simulink model "ieee9bus_wind_farm"  (R2015b)
settings: Solver=FixedStepAuto  StartTime=0.0  StopTime=40  FixedStep=Ts  RelTol=1e-3
values from neighbouring files (symbols this model uses):
  Cbase = 1/(100*pi*Xbase)    (= 6.0172001169e-06)    [ieee_9.m]
  Lbase = Xbase/(100*pi)    (= 1.68385929791)    [ieee_9.m]
  loadconnection = 15    [ieee_9.m]
  startup = 2    [ieee_9.m]
  Ts = 1e-5    (= 1e-05)    [ieee_9.m]
  Xbase = (Vbase^2)/Sbase    (= 529)    [ieee_9.m]
libraries: powerlib x125, powerlib_meascontrol x23, simulink x10, sps_avr x4, powerlib_extras x1
(part 2 of 2)

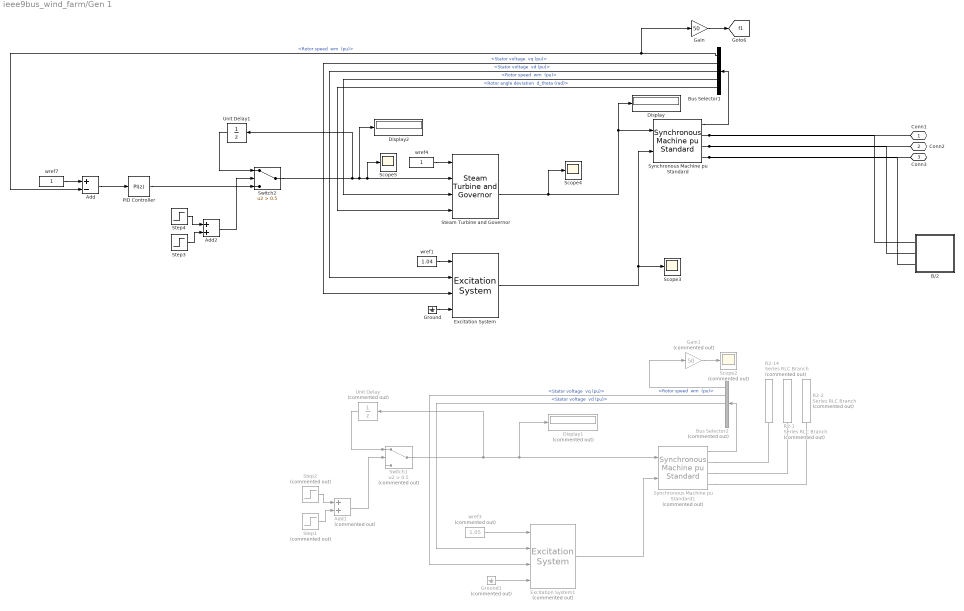
== system ieee9bus_wind_farm/Gen 1 ==
  Add : Sum  Inputs=+-
  Add1 : Sum  Commented=on
  Add2 : Sum
  B/2 : Subsystem
  Bus Selector1 : BusSelector  OutputSignals="Mechanical.Rotor speed  wm  (pu),dq0 components.Stator voltage  vq (pu),dq0 components.Stator voltage  vd (pu),Mechanical.Rotor speed  wm  (pu),Mechanical.Rotor angle deviation  d_theta (rad)"
  Bus Selector2 : BusSelector  Commented=on  OutputSignals="Mechanical.Rotor speed  wm  (pu),dq0 components.Stator voltage  vq (pu),dq0 components.Stator voltage  vd (pu),Mechanical.Rotor speed  wm  (pu),Mechanical.Rotor angle deviation  d_theta (rad)"
  Display : Display
  Display1 : Display  Commented=on
  Display2 : Display
  Excitation System : sps_avr/Excitation System  tr=20e-3  reg=[ 350, 0.001 ]  exc=[ 1, 0 ]  tgr=[ 0, 0 ]  damp=[ 0.001, 0.1 ]  sat=[ 0, 0 ]  lim=[ -11.5, 11.5, 0 ]  v0="[1.0  1.28]"
  Excitation System1 : sps_avr/Excitation System  Commented=on  tr=20e-3  reg=[ 350, 0.001 ]  exc=[ 1, 0 ]  tgr=[ 0, 0 ]  damp=[ 0.001, 0.1 ]  sat=[ 0, 0 ]  lim=[ -11.5, 11.5, 0 ]  v0="[1.0  1.28]"
  Gain : Gain  Gain=50
  Gain1 : Gain  Commented=on  Gain=50
  Ground : Ground
  Ground1 : Ground  Commented=on
  PID Controller : simulink/Continuous/PID Controller  Controller=PI  TimeDomain=Discrete-time  SampleTime=Ts  IntegratorMethod=Forward Euler  FilterMethod=Forward Euler  Form=Parallel  UseFilter=on  ControllerParametersSource=internal  P=1  I=2.5  D=0  N=100  InitialConditionSource=internal  InitialConditionForIntegrator=70/247.5  InitialConditionForFilter=0  ExternalReset=none  LimitOutput=on  UpperSaturationLimit=1  LowerSaturationLimit=1e-6  LinearizeAsGain=on  AntiWindupMode=none  Kb=1  TrackingMode=off  Kt=1  PParamMin=[]  PParamMax=[]  IParamMin=[]  IParamMax=[]  DParamMin=[]  DParamMax=[]  NParamMin=[]  NParamMax=[]  KbParamMin=[]  KbParamMax=[]  KtParamMin=[]  KtParamMax=[]  POutMin=[]  POutMax=[]  IOutMin=[]  IOutMax=[]  DOutMin=[]  DOutMax=[]  NOutMin=[]  NOutMax=[]  KbOutMin=[]  KbOutMax=[]  KtOutMin=[]  KtOutMax=[]  IntegratorOutMin=[]  IntegratorOutMax=[]  FilterOutMin=[]  FilterOutMax=[]  SumOutMin=[]  SumOutMax=[]  SumI1OutMin=[]  SumI1OutMax=[]  SumI2OutMin=[]  SumI2OutMax=[]  SumI3OutMin=[]  SumI3OutMax=[]  SumDOutMin=[]  SumDOutMax=[]  SaturationOutMin=[]  SaturationOutMax=[]  IntegratorContinuousStateAttributes=''  IntegratorStateMustResolveToSignalObject=off  IntegratorRTWStateStorageClass=Auto  FilterContinuousStateAttributes=''  FilterStateMustResolveToSignalObject=off  FilterRTWStateStorageClass=Auto  DifferentiatorICPrevScaledInput=0  DifferentiatorOutMin=[]  DifferentiatorOutMax=[]
  R2-1 : powerlib/Elements/Series RLC Branch  Commented=on  LConnTagsString=__new0  RConnTagsString=__new0  BranchType=R  Resistance=0.0000001  Inductance=0.3*Xbase  SetiL0=off  InitialCurrent=0  Capacitance=1e-6  Setx0=off  InitialVoltage=0  Measurements=None
  R2-14 : powerlib/Elements/Series RLC Branch  Commented=on  LConnTagsString=__new0  RConnTagsString=__new0  BranchType=R  Resistance=0.0000001  Inductance=0.3*Xbase  SetiL0=off  InitialCurrent=0  Capacitance=1e-6  Setx0=off  InitialVoltage=0  Measurements=None
  R2-2 : powerlib/Elements/Series RLC Branch  Commented=on  LConnTagsString=__new0  RConnTagsString=__new0  BranchType=R  Resistance=0.0000001  Inductance=0.3*Xbase  SetiL0=off  InitialCurrent=0  Capacitance=1e-6  Setx0=off  InitialVoltage=0  Measurements=None
  Scope2 : Scope  Commented=on
  Scope3 : Scope
  Scope4 : Scope
  Scope5 : Scope
  Steam Turbine and Governor : powerlib/Machines/Steam Turbine and Governor  gentype=Tandem-compound (multi-mass)  reg1="[ 1  0.05    0 ]"  reg2="[ 0.001  0.3 ]"  reg3="[ -0.1  0.1  0  4.496]"  N=1500  turb1="[ 0  10   3.3   0.5   ]"  turb2="[ 0.5   0.5   0  0 ]"  HA="[  1.5498   0.24894  0  0 ]"  KA="[  83.47  42.702  0  0 ]"  DA="[  0.3104  0.05  0  0 ]*8"  ini1=250.35/555  ini2=[0.5,-120.13]
  Step1 : Step  Commented=on  Time=loadconnection-1  SampleTime=Ts
  Step2 : Step  Commented=on  Time=startup  Before=1  After=0  SampleTime=Ts
  Step3 : Step  Time=loadconnection-1  SampleTime=Ts
  Step4 : Step  Time=startup-2  Before=1  After=0  SampleTime=Ts
  Switch1 : Switch  Commented=on  Criteria=u2 > Threshold  Threshold=0.5
  Switch2 : Switch  Criteria=u2 > Threshold  Threshold=0.5
  Synchronous Machine pu Standard : powerlib/Machines/Synchronous Machine pu Standard  PresetModel=No  MechanicalLoad=Mechanical power Pm  ShowDetailedParameters=on  RotorType=Salient-pole  Units=per unit standard parameters  MeasurementBus=off  NominalParameters=[247.5e+06 16.5e3 50]  Reactances1=[ 1.81, 0.15048, 0.1, 1.76, 0.65, 0.25, 0.15 ]  Reactances2=[0.36135 0.15048 0.1 0.2398275 0.1 0.08316]  dAxisTimeConstants=Short-circuit  qAxisTimeConstants=Short-circuit  TimeConstants1="[ 4.4849  0.0681  0.1  ]"  TimeConstants2=[ 8.0, 0.03, 1.0, 0.07 ]  TimeConstants3="[  4.49  0.0681  0.0513  ]"  TimeConstants4=[ 8.0, 0.03, 0.3371, 0.0295 ]  TimeConstants5=[ 1.01, 0.053, 0.1 ]  TimeConstants6=[ 1.3201, 0.023, 1.0, 0.07 ]  TimeConstants7=[8.96 0.075 0.15]  TimeConstants8=[ 1.3201, 0.0231, 0.3371, 0.0295 ]  StatorResistance=0.00000001  Mechanical=[9.55 0.02056 4]  PolePairs=20  InitialConditions="[ 0  0  0  0  0  0  0  0  1 ]"  SetSaturation=off  Saturation=[0.6404,0.7127,0.8441,0.9214,0.9956,1.082,1.19,1.316,1.457;0.7,0.7698,0.8872,0.9466,0.9969,1.046,1.1,1.151,1.201]  LoadFlowParameters=[1,0,0,0,0]  TsPowergui=0  TsBlock=-1  IterativeModel=Trapezoidal non iterative  BusType=swing  Pref=0  Qref=0  Qmin=-inf  Qmax=inf  PLF=0  QLF=0
  Synchronous Machine pu Standard1 : powerlib/Machines/Synchronous Machine pu Standard  Commented=on  PresetModel=No  MechanicalLoad=Mechanical power Pm  ShowDetailedParameters=on  RotorType=Round  Units=per unit standard parameters  MeasurementBus=off  NominalParameters=[25e+06 16.5e3 50]  Reactances1=[ 1.81, 0.3, 0.23, 1.76, 0.65, 0.25, 0.15 ]  Reactances2=[2.24 0.17 0.12 1.02 0.13 0.08]  dAxisTimeConstants=Short-circuit  qAxisTimeConstants=Short-circuit  TimeConstants1="[ 4.4849  0.0681  0.1  ]"  TimeConstants2=[ 8.0, 0.03, 1.0, 0.07 ]  TimeConstants3="[  4.49  0.0681  0.0513  ]"  TimeConstants4=[ 8.0, 0.03, 0.3371, 0.0295 ]  TimeConstants5=[ 1.01, 0.053, 0.1 ]  TimeConstants6=[ 1.3201, 0.023, 1.0, 0.07 ]  TimeConstants7=[0.012 0.003 0.003]  TimeConstants8=[ 1.3201, 0.0231, 0.3371, 0.0295 ]  StatorResistance=0.0000107875  Mechanical=[2 0.02056 4]  PolePairs=20  InitialConditions="[ 0  0  0  0  0  0  0  0  1 ]"  SetSaturation=off  Saturation=[0.6404,0.7127,0.8441,0.9214,0.9956,1.082,1.19,1.316,1.457;0.7,0.7698,0.8872,0.9466,0.9969,1.046,1.1,1.151,1.201]  LoadFlowParameters=[1,0,0,0,0]  TsPowergui=0  TsBlock=-1  IterativeModel=Trapezoidal non iterative  BusType=swing  Pref=0  Qref=0  Qmin=-inf  Qmax=inf  PLF=0  QLF=0
  Unit Delay : UnitDelay  Commented=on  SampleTime=Ts
  Unit Delay1 : UnitDelay  SampleTime=Ts
  wref1 : Constant  Value=1.04
  wref3 : Constant  Commented=on  Value=1.05
  wref4 : Constant
  wref7 : Constant
  Conn1 : PMIOPort  Port=1  Side=Right
  Conn2 : PMIOPort  Port=2  Side=Right
  Conn3 : PMIOPort  Port=3  Side=Right
  tag scope: f1=global
  wires:
  Synchronous Machine pu Standard/1 -> Bus Selector1/1
  wref1/1 -> Excitation System/1
  Ground/1 -> Excitation System/4
  Excitation System/1 -> Synchronous Machine pu Standard/2, Scope3/1
  Bus Selector1/3 -> Excitation System/2  "<Stator voltage  vd (pu)>"
  Bus Selector1/1 -> Add/2, Gain/1  "<Rotor speed  wm  (pu)>"
  Bus Selector1/2 -> Excitation System/3  "<Stator voltage  vq (pu)>"
  Gain/1 -> [f1]
  Bus Selector1/4 -> Steam Turbine and Governor/3  "<Rotor speed  wm  (pu)>"
  wref4/1 -> Steam Turbine and Governor/1
  Bus Selector1/5 -> Steam Turbine and Governor/4  "<Rotor angle deviation  d_theta (rad)>"
  Steam Turbine and Governor/3 -> Scope4/1, Display/1, Synchronous Machine pu Standard/1
  Synchronous Machine pu Standard1/1 -> Bus Selector2/1
  wref3/1 -> Excitation System1/1
  Ground1/1 -> Excitation System1/4
  Excitation System1/1 -> Synchronous Machine pu Standard1/2
  Bus Selector2/3 -> Excitation System1/2  "<Stator voltage  vd (pu)>"
  Bus Selector2/1 -> Gain1/1  "<Rotor speed  wm  (pu)>"
  Bus Selector2/2 -> Excitation System1/3  "<Stator voltage  vq (pu)>"
  Gain1/1 -> Scope2/1
  Switch1/1 -> Unit Delay/1, Display1/1, Synchronous Machine pu Standard1/1
  Unit Delay/1 -> Switch1/1
  wref7/1 -> Add/1
  Add/1 -> PID Controller/1
  Step2/1 -> Add1/1
  Step1/1 -> Add1/2
  Add1/1 -> Switch1/2
  Switch2/1 -> Display2/1, Scope5/1, Steam Turbine and Governor/2, Unit Delay1/1
  Unit Delay1/1 -> Switch2/1
  PID Controller/1 -> Switch2/3
  Step4/1 -> Add2/1
  Step3/1 -> Add2/2
  Add2/1 -> Switch2/2
  connections:
  Synchronous Machine pu Standard1/RConn3 -- R2-2/RConn1
  Synchronous Machine pu Standard1/RConn2 -- R2-1/RConn1
  Synchronous Machine pu Standard1/RConn1 -- R2-14/RConn1
  Synchronous Machine pu Standard/RConn3 -- Conn3/RConn1 -- B/2/RConn3
  Synchronous Machine pu Standard/RConn2 -- Conn2/RConn1 -- B/2/RConn2
  Synchronous Machine pu Standard/RConn1 -- Conn1/RConn1 -- B/2/RConn1

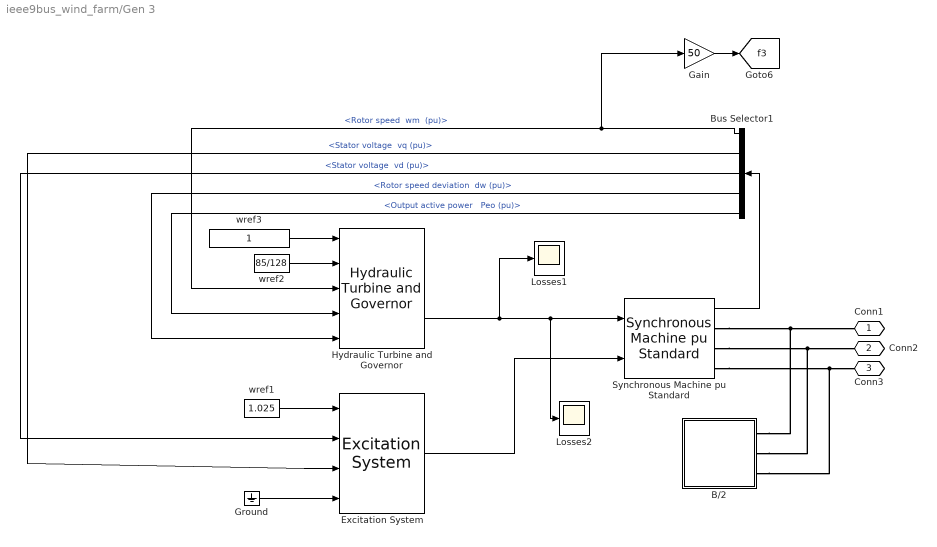
== system ieee9bus_wind_farm/Gen 3 ==
  B/2 : Subsystem
  Bus Selector1 : BusSelector  OutputSignals="Mechanical.Rotor speed  wm  (pu),dq0 components.Stator voltage  vq (pu),dq0 components.Stator voltage  vd (pu),Mechanical.Rotor speed deviation  dw (pu),Output active power   Peo (pu)"
  Excitation System : sps_avr/Excitation System  tr=20e-3  reg=[ 350, 0.001 ]  exc=[ 1, 0 ]  tgr=[ 0, 0 ]  damp=[ 0.001, 0.1 ]  sat=[ 0, 0 ]  lim=[ -11.5, 11.5, 0 ]  v0="[1.0  1.28]"
  Gain : Gain  Gain=50
  Ground : Ground
  Hydraulic Turbine and Governor : powerlib/Machines/Hydraulic Turbine and Governor  sm="[ 10/3  0.07 ]"  gate="[  0.01  0.97518  -0.1  0.1 ]"  reg="[  0.05  1.163  0.105  0  0.01  ]"  hyd="[  0  2.67  ]"  dref=0  po=90/128
  Losses1 : Scope
  Losses2 : Scope
  Synchronous Machine pu Standard : powerlib/Machines/Synchronous Machine pu Standard  PresetModel=No  MechanicalLoad=Mechanical power Pm  ShowDetailedParameters=on  RotorType=Round  Units=per unit standard parameters  MeasurementBus=off  NominalParameters=[128e+06 13.8e3 50]  Reactances1=[ 1.68, 0.232064, 0.2, 1.609984, 0.32, 0.2, 0.094976 ]  Reactances2=[2.24 0.17 0.12 1.02 0.13 0.08]  dAxisTimeConstants=Short-circuit  qAxisTimeConstants=Short-circuit  TimeConstants1="[ 4.4849  0.0681  0.1  ]"  TimeConstants2=[ 8.0, 0.03, 1.0, 0.07 ]  TimeConstants3="[  4.49  0.0681  0.0513  ]"  TimeConstants4=[ 8.0, 0.03, 0.3371, 0.0295 ]  TimeConstants5=[ 1.01, 0.053, 0.1 ]  TimeConstants6=[ 1.3201, 0.023, 1.0, 0.07 ]  TimeConstants7=[0.012 0.003 0.003]  TimeConstants8=[ 5.89, 0.0575, 0.6, 0.08 ]  StatorResistance=0.0000000107875  Mechanical=[2.35 0.02056 4]  PolePairs=20  InitialConditions="[ 0  0  0  0  0  0  0  0  1 ]"  SetSaturation=off  Saturation=[0.6404,0.7127,0.8441,0.9214,0.9956,1.082,1.19,1.316,1.457;0.7,0.7698,0.8872,0.9466,0.9969,1.046,1.1,1.151,1.201]  LoadFlowParameters=[1,0,0,0,0]  TsPowergui=0  TsBlock=-1  IterativeModel=Trapezoidal non iterative  BusType=swing  Pref=50e6  Qref=0  Qmin=-inf  Qmax=inf  PLF=0  QLF=0
  wref1 : Constant  Value=1.025
  wref2 : Constant  Value=85/128
  wref3 : Constant
  Conn1 : PMIOPort  Port=1  Side=Right
  Conn2 : PMIOPort  Port=2  Side=Right
  Conn3 : PMIOPort  Port=3  Side=Right
  tag scope: f3=global
  wires:
  Gain/1 -> [f3]
  Bus Selector1/2 -> Excitation System/3  "<Stator voltage  vq (pu)>"
  Bus Selector1/1 -> Hydraulic Turbine and Governor/3, Gain/1  "<Rotor speed  wm  (pu)>"
  Bus Selector1/3 -> Excitation System/2  "<Stator voltage  vd (pu)>"
  Excitation System/1 -> Synchronous Machine pu Standard/2
  Ground/1 -> Excitation System/4
  wref1/1 -> Excitation System/1
  Synchronous Machine pu Standard/1 -> Bus Selector1/1
  wref3/1 -> Hydraulic Turbine and Governor/1
  Bus Selector1/4 -> Hydraulic Turbine and Governor/5  "<Rotor speed deviation  dw (pu)>"
  Bus Selector1/5 -> Hydraulic Turbine and Governor/4  "<Output active power   Peo (pu)>"
  wref2/1 -> Hydraulic Turbine and Governor/2
  Hydraulic Turbine and Governor/2 -> Losses1/1, Losses2/1, Synchronous Machine pu Standard/1
  connections:
  Synchronous Machine pu Standard/RConn1 -- Conn1/RConn1 -- B/2/RConn1
  Synchronous Machine pu Standard/RConn2 -- Conn2/RConn1 -- B/2/RConn2
  Synchronous Machine pu Standard/RConn3 -- Conn3/RConn1 -- B/2/RConn3

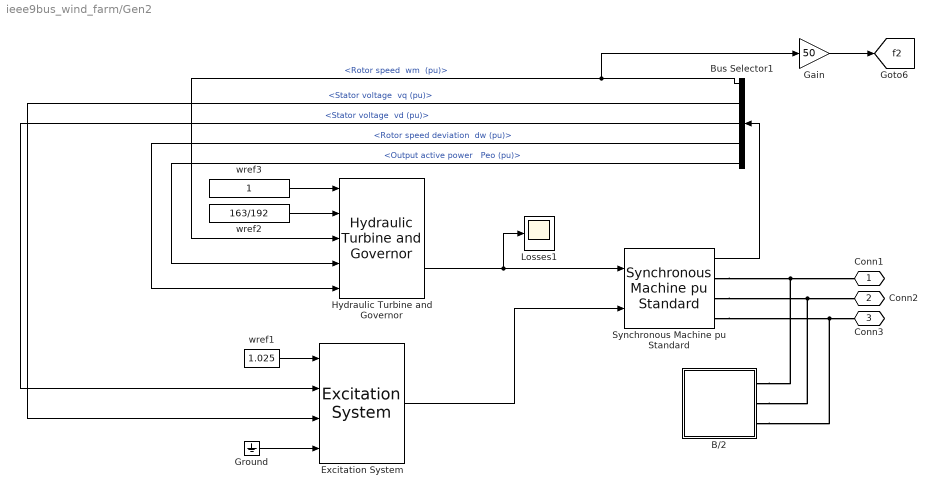
== system ieee9bus_wind_farm/Gen2 ==
  B/2 : Subsystem
  Bus Selector1 : BusSelector  OutputSignals="Mechanical.Rotor speed  wm  (pu),dq0 components.Stator voltage  vq (pu),dq0 components.Stator voltage  vd (pu),Mechanical.Rotor speed deviation  dw (pu),Output active power   Peo (pu)"
  Excitation System : sps_avr/Excitation System  tr=20e-3  reg=[ 350, 0.001 ]  exc=[ 1, 0 ]  tgr=[ 0, 0 ]  damp=[ 0.001, 0.1 ]  sat=[ 0, 0 ]  lim=[ -11.5, 11.5, 0 ]  v0="[1.0  1.28]"
  Gain : Gain  Gain=50
  Ground : Ground
  Hydraulic Turbine and Governor : powerlib/Machines/Hydraulic Turbine and Governor  sm="[ 10/3  0.07 ]"  gate="[  0.01  0.97518  -0.1  0.1 ]"  reg="[  0.05  1.163  0.105  0  0.01  ]"  hyd="[  0  2.67  ]"  dref=0  po=170/192
  Losses1 : Scope
  Synchronous Machine pu Standard : powerlib/Machines/Synchronous Machine pu Standard  PresetModel=No  MechanicalLoad=Mechanical power Pm  ShowDetailedParameters=on  RotorType=Round  Units=per unit standard parameters  MeasurementBus=off  NominalParameters=[192e+06 18e3 50]  Reactances1=[1.719936 0.230016 0.2 1.65984 0.378048 0.2 0.100032]  Reactances2=[1.719936 0.230016 0.2 1.65984 0.100032]  dAxisTimeConstants=Short-circuit  qAxisTimeConstants=Short-circuit  TimeConstants1="[ 4.4849  0.0681  0.1  ]"  TimeConstants2=[ 8.0, 0.03, 1.0, 0.07 ]  TimeConstants3="[  4.49  0.0681  0.0513  ]"  TimeConstants4=[ 8.0, 0.03, 0.3371, 0.0295 ]  TimeConstants5=[ 1.01, 0.053, 0.1 ]  TimeConstants6=[ 1.3201, 0.023, 1.0, 0.07 ]  TimeConstants7=[6 0.0575 0.0945]  TimeConstants8=[ 6 0.0575 0.535 0.0945]  StatorResistance=0.005  Mechanical=[3.33 0.02056 4]  PolePairs=20  InitialConditions="[ 0  0  0  0  0  0  0  0  1 ]"  SetSaturation=off  Saturation=[0.6404,0.7127,0.8441,0.9214,0.9956,1.082,1.19,1.316,1.457;0.7,0.7698,0.8872,0.9466,0.9969,1.046,1.1,1.151,1.201]  LoadFlowParameters=[1,0,0,0,0]  TsPowergui=0  TsBlock=-1  IterativeModel=Trapezoidal non iterative  BusType=swing  Pref=50e6  Qref=0  Qmin=-inf  Qmax=inf  PLF=0  QLF=0
  wref1 : Constant  Value=1.025
  wref2 : Constant  Value=163/192
  wref3 : Constant
  Conn1 : PMIOPort  Port=1  Side=Right
  Conn2 : PMIOPort  Port=2  Side=Right
  Conn3 : PMIOPort  Port=3  Side=Right
  tag scope: f2=global
  wires:
  Hydraulic Turbine and Governor/2 -> Losses1/1, Synchronous Machine pu Standard/1
  Gain/1 -> [f2]
  Bus Selector1/2 -> Excitation System/3  "<Stator voltage  vq (pu)>"
  Bus Selector1/1 -> Hydraulic Turbine and Governor/3, Gain/1  "<Rotor speed  wm  (pu)>"
  Bus Selector1/3 -> Excitation System/2  "<Stator voltage  vd (pu)>"
  Excitation System/1 -> Synchronous Machine pu Standard/2
  Ground/1 -> Excitation System/4
  wref1/1 -> Excitation System/1
  Synchronous Machine pu Standard/1 -> Bus Selector1/1
  wref3/1 -> Hydraulic Turbine and Governor/1
  Bus Selector1/4 -> Hydraulic Turbine and Governor/5  "<Rotor speed deviation  dw (pu)>"
  Bus Selector1/5 -> Hydraulic Turbine and Governor/4  "<Output active power   Peo (pu)>"
  wref2/1 -> Hydraulic Turbine and Governor/2
  connections:
  Synchronous Machine pu Standard/RConn1 -- Conn1/RConn1 -- B/2/RConn1
  Synchronous Machine pu Standard/RConn2 -- Conn2/RConn1 -- B/2/RConn2
  Synchronous Machine pu Standard/RConn3 -- Conn3/RConn1 -- B/2/RConn3

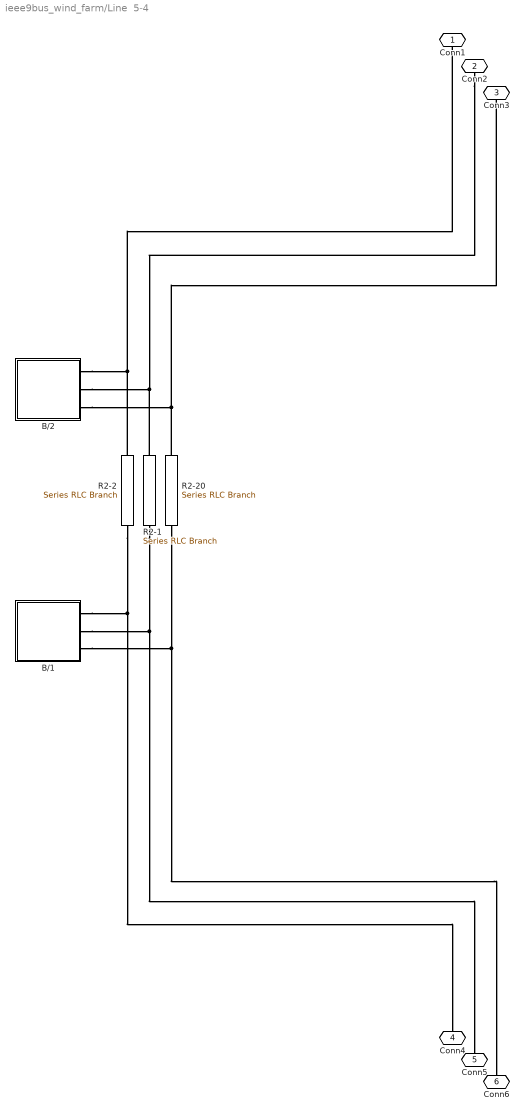
== system ieee9bus_wind_farm/Line  5-4 ==
  B/1 : Subsystem
  B/2 : Subsystem
  R2-1 : powerlib/Elements/Series RLC Branch  LConnTagsString=__new0  RConnTagsString=__new0  BranchType=RL  Resistance=0.01*Xbase  Inductance=0.085*Lbase  SetiL0=off  InitialCurrent=0  Capacitance=1e-6  Setx0=off  InitialVoltage=0  Measurements=None
  R2-2 : powerlib/Elements/Series RLC Branch  LConnTagsString=__new0  RConnTagsString=__new0  BranchType=RL  Resistance=0.01*Xbase  Inductance=0.085*Lbase  SetiL0=off  InitialCurrent=0  Capacitance=1e-6  Setx0=off  InitialVoltage=0  Measurements=None
  R2-20 : powerlib/Elements/Series RLC Branch  LConnTagsString=__new0  RConnTagsString=__new0  BranchType=RL  Resistance=0.01*Xbase  Inductance=0.085*Lbase  SetiL0=off  InitialCurrent=0  Capacitance=1e-6  Setx0=off  InitialVoltage=0  Measurements=None
  Conn1 : PMIOPort  Port=1  Side=Right
  Conn2 : PMIOPort  Port=2  Side=Right
  Conn3 : PMIOPort  Port=3  Side=Right
  Conn4 : PMIOPort  Port=4  Side=Left
  Conn5 : PMIOPort  Port=5  Side=Left
  Conn6 : PMIOPort  Port=6  Side=Left
  connections:
  B/1/RConn1 -- Conn4/RConn1 -- R2-2/RConn1
  R2-20/RConn1 -- Conn6/RConn1 -- B/1/RConn3
  Conn2/RConn1 -- R2-1/LConn1 -- B/2/RConn2
  B/2/RConn1 -- R2-2/LConn1 -- Conn1/RConn1
  R2-20/LConn1 -- B/2/RConn3 -- Conn3/RConn1
  B/1/RConn2 -- Conn5/RConn1 -- R2-1/RConn1

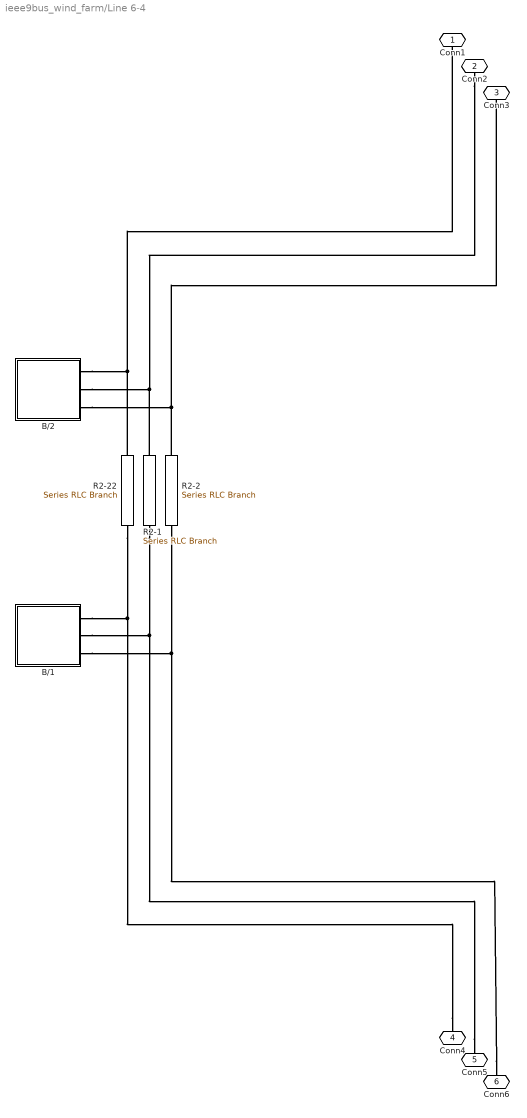
== system ieee9bus_wind_farm/Line 6-4 ==
  B/1 : Subsystem
  B/2 : Subsystem
  R2-1 : powerlib/Elements/Series RLC Branch  LConnTagsString=__new0  RConnTagsString=__new0  BranchType=RL  Resistance=0.017*Xbase  Inductance=0.092*Lbase  SetiL0=off  InitialCurrent=0  Capacitance=1e-6  Setx0=off  InitialVoltage=0  Measurements=None
  R2-2 : powerlib/Elements/Series RLC Branch  LConnTagsString=__new0  RConnTagsString=__new0  BranchType=RL  Resistance=0.017*Xbase  Inductance=0.092*Lbase  SetiL0=off  InitialCurrent=0  Capacitance=1e-6  Setx0=off  InitialVoltage=0  Measurements=None
  R2-22 : powerlib/Elements/Series RLC Branch  LConnTagsString=__new0  RConnTagsString=__new0  BranchType=RL  Resistance=0.017*Xbase  Inductance=0.092*Lbase  SetiL0=off  InitialCurrent=0  Capacitance=1e-6  Setx0=off  InitialVoltage=0  Measurements=None
  Conn1 : PMIOPort  Port=1  Side=Right
  Conn2 : PMIOPort  Port=2  Side=Right
  Conn3 : PMIOPort  Port=3  Side=Right
  Conn4 : PMIOPort  Port=4  Side=Left
  Conn5 : PMIOPort  Port=5  Side=Left
  Conn6 : PMIOPort  Port=6  Side=Left
  connections:
  Conn5/RConn1 -- B/1/RConn2 -- R2-1/RConn1
  Conn3/RConn1 -- R2-2/LConn1 -- B/2/RConn3
  Conn1/RConn1 -- B/2/RConn1 -- R2-22/LConn1
  B/2/RConn2 -- R2-1/LConn1 -- Conn2/RConn1
  Conn6/RConn1 -- B/1/RConn3 -- R2-2/RConn1
  Conn4/RConn1 -- B/1/RConn1 -- R2-22/RConn1

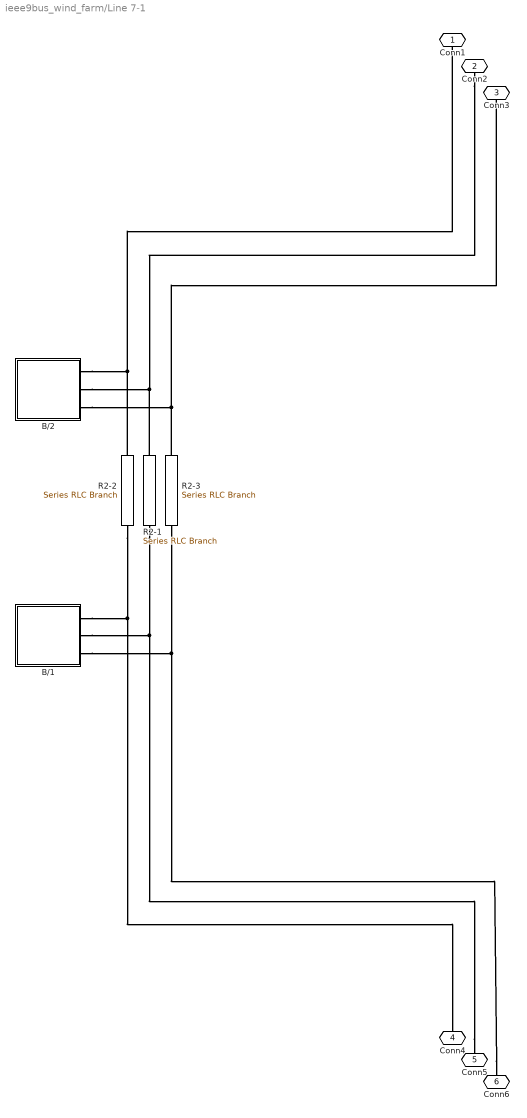
== system ieee9bus_wind_farm/Line 7-1 ==
  B/1 : Subsystem
  B/2 : Subsystem
  R2-1 : powerlib/Elements/Series RLC Branch  LConnTagsString=__new0  RConnTagsString=__new0  BranchType=RL  Resistance=0.0119*Xbase  Inductance=0.1008*Lbase  SetiL0=off  InitialCurrent=0  Capacitance=1e-6  Setx0=off  InitialVoltage=0  Measurements=None
  R2-2 : powerlib/Elements/Series RLC Branch  LConnTagsString=__new0  RConnTagsString=__new0  BranchType=RL  Resistance=0.0119*Xbase  Inductance=0.1008*Lbase  SetiL0=off  InitialCurrent=0  Capacitance=1e-6  Setx0=off  InitialVoltage=0  Measurements=None
  R2-3 : powerlib/Elements/Series RLC Branch  LConnTagsString=__new0  RConnTagsString=__new0  BranchType=RL  Resistance=0.0119*Xbase  Inductance=0.1008*Lbase  SetiL0=off  InitialCurrent=0  Capacitance=1e-6  Setx0=off  InitialVoltage=0  Measurements=None
  Conn1 : PMIOPort  Port=1  Side=Right
  Conn2 : PMIOPort  Port=2  Side=Right
  Conn3 : PMIOPort  Port=3  Side=Right
  Conn4 : PMIOPort  Port=4  Side=Left
  Conn5 : PMIOPort  Port=5  Side=Left
  Conn6 : PMIOPort  Port=6  Side=Left
  connections:
  Conn5/RConn1 -- B/1/RConn2 -- R2-1/RConn1
  Conn3/RConn1 -- R2-3/LConn1 -- B/2/RConn3
  Conn1/RConn1 -- R2-2/LConn1 -- B/2/RConn1
  B/2/RConn2 -- R2-1/LConn1 -- Conn2/RConn1
  Conn6/RConn1 -- B/1/RConn3 -- R2-3/RConn1
  R2-2/RConn1 -- B/1/RConn1 -- Conn4/RConn1

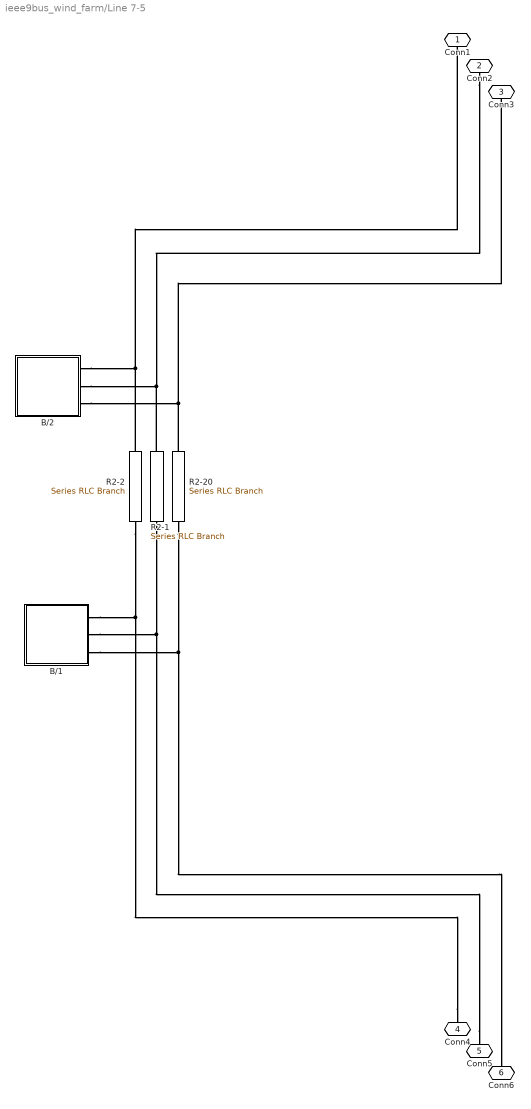
== system ieee9bus_wind_farm/Line 7-5 ==
  B/1 : Subsystem
  B/2 : Subsystem
  R2-1 : powerlib/Elements/Series RLC Branch  LConnTagsString=__new0  RConnTagsString=__new0  BranchType=RL  Resistance=0.0032*Xbase  Inductance=0.161*Lbase  SetiL0=off  InitialCurrent=0  Capacitance=1e-6  Setx0=off  InitialVoltage=0  Measurements=None
  R2-2 : powerlib/Elements/Series RLC Branch  LConnTagsString=__new0  RConnTagsString=__new0  BranchType=RL  Resistance=0.0032*Xbase  Inductance=0.161*Lbase  SetiL0=off  InitialCurrent=0  Capacitance=1e-6  Setx0=off  InitialVoltage=0  Measurements=None
  R2-20 : powerlib/Elements/Series RLC Branch  LConnTagsString=__new0  RConnTagsString=__new0  BranchType=RL  Resistance=0.0032*Xbase  Inductance=0.161*Lbase  SetiL0=off  InitialCurrent=0  Capacitance=1e-6  Setx0=off  InitialVoltage=0  Measurements=None
  Conn1 : PMIOPort  Port=1  Side=Right
  Conn2 : PMIOPort  Port=2  Side=Right
  Conn3 : PMIOPort  Port=3  Side=Right
  Conn4 : PMIOPort  Port=4  Side=Left
  Conn5 : PMIOPort  Port=5  Side=Left
  Conn6 : PMIOPort  Port=6  Side=Left
  connections:
  Conn4/RConn1 -- B/1/RConn1 -- R2-2/RConn1
  R2-20/RConn1 -- B/1/RConn3 -- Conn6/RConn1
  Conn2/RConn1 -- B/2/RConn2 -- R2-1/LConn1
  R2-2/LConn1 -- B/2/RConn1 -- Conn1/RConn1
  R2-20/LConn1 -- B/2/RConn3 -- Conn3/RConn1
  Conn5/RConn1 -- B/1/RConn2 -- R2-1/RConn1

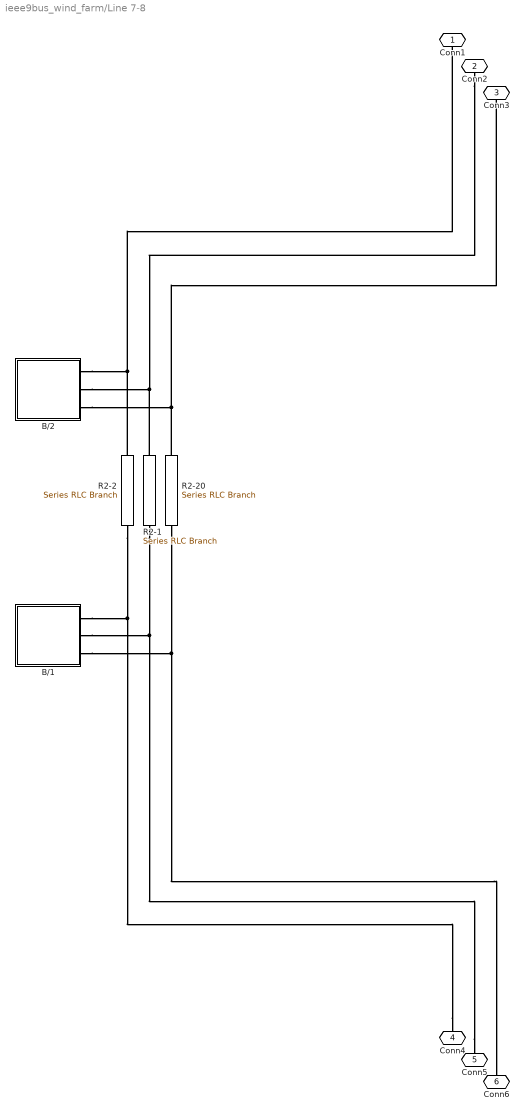
== system ieee9bus_wind_farm/Line 7-8 ==
  B/1 : Subsystem
  B/2 : Subsystem
  R2-1 : powerlib/Elements/Series RLC Branch  LConnTagsString=__new0  RConnTagsString=__new0  BranchType=RL  Resistance=0.0085*Xbase  Inductance=0.072*Lbase  SetiL0=off  InitialCurrent=0  Capacitance=1e-6  Setx0=off  InitialVoltage=0  Measurements=None
  R2-2 : powerlib/Elements/Series RLC Branch  LConnTagsString=__new0  RConnTagsString=__new0  BranchType=RL  Resistance=0.0085*Xbase  Inductance=0.072*Lbase  SetiL0=off  InitialCurrent=0  Capacitance=1e-6  Setx0=off  InitialVoltage=0  Measurements=None
  R2-20 : powerlib/Elements/Series RLC Branch  LConnTagsString=__new0  RConnTagsString=__new0  BranchType=RL  Resistance=0.0085*Xbase  Inductance=0.072*Lbase  SetiL0=off  InitialCurrent=0  Capacitance=1e-6  Setx0=off  InitialVoltage=0  Measurements=None
  Conn1 : PMIOPort  Port=1  Side=Right
  Conn2 : PMIOPort  Port=2  Side=Right
  Conn3 : PMIOPort  Port=3  Side=Right
  Conn4 : PMIOPort  Port=4  Side=Left
  Conn5 : PMIOPort  Port=5  Side=Left
  Conn6 : PMIOPort  Port=6  Side=Left
  connections:
  Conn4/RConn1 -- B/1/RConn1 -- R2-2/RConn1
  R2-20/RConn1 -- B/1/RConn3 -- Conn6/RConn1
  Conn2/RConn1 -- R2-1/LConn1 -- B/2/RConn2
  B/2/RConn1 -- R2-2/LConn1 -- Conn1/RConn1
  R2-20/LConn1 -- B/2/RConn3 -- Conn3/RConn1
  Conn5/RConn1 -- B/1/RConn2 -- R2-1/RConn1

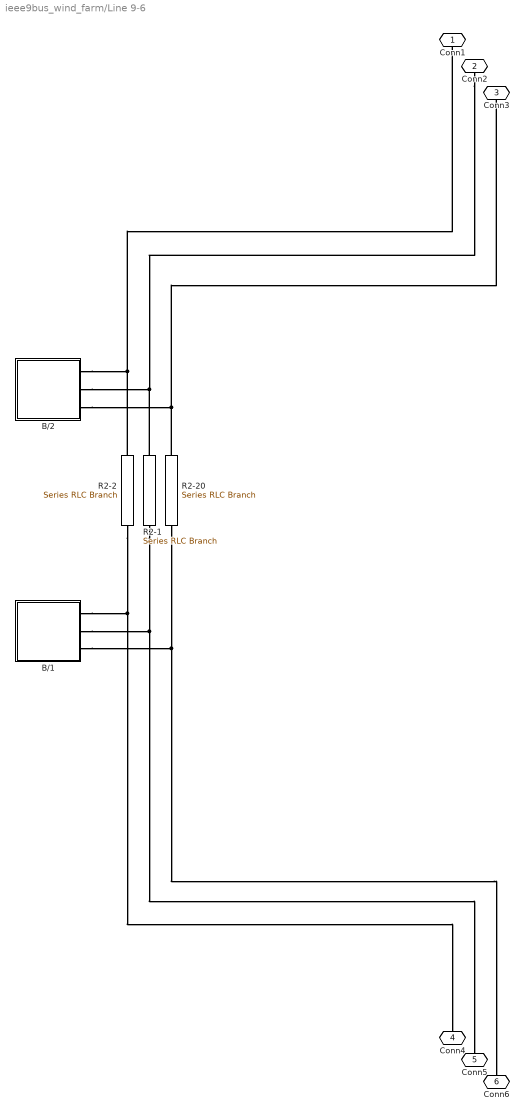
== system ieee9bus_wind_farm/Line 9-6 ==
  B/1 : Subsystem
  B/2 : Subsystem
  R2-1 : powerlib/Elements/Series RLC Branch  LConnTagsString=__new0  RConnTagsString=__new0  BranchType=RL  Resistance=0.039*Xbase  Inductance=0.17*Lbase  SetiL0=off  InitialCurrent=0  Capacitance=1e-6  Setx0=off  InitialVoltage=0  Measurements=None
  R2-2 : powerlib/Elements/Series RLC Branch  LConnTagsString=__new0  RConnTagsString=__new0  BranchType=RL  Resistance=0.039*Xbase  Inductance=0.17*Lbase  SetiL0=off  InitialCurrent=0  Capacitance=1e-6  Setx0=off  InitialVoltage=0  Measurements=None
  R2-20 : powerlib/Elements/Series RLC Branch  LConnTagsString=__new0  RConnTagsString=__new0  BranchType=RL  Resistance=0.039*Xbase  Inductance=0.17*Lbase  SetiL0=off  InitialCurrent=0  Capacitance=1e-6  Setx0=off  InitialVoltage=0  Measurements=None
  Conn1 : PMIOPort  Port=1  Side=Right
  Conn2 : PMIOPort  Port=2  Side=Right
  Conn3 : PMIOPort  Port=3  Side=Right
  Conn4 : PMIOPort  Port=4  Side=Left
  Conn5 : PMIOPort  Port=5  Side=Left
  Conn6 : PMIOPort  Port=6  Side=Left
  connections:
  B/1/RConn2 -- Conn5/RConn1 -- R2-1/RConn1
  Conn3/RConn1 -- B/2/RConn3 -- R2-20/LConn1
  Conn1/RConn1 -- R2-2/LConn1 -- B/2/RConn1
  B/2/RConn2 -- R2-1/LConn1 -- Conn2/RConn1
  B/1/RConn3 -- Conn6/RConn1 -- R2-20/RConn1
  B/1/RConn1 -- Conn4/RConn1 -- R2-2/RConn1

== system ieee9bus_wind_farm/GE2.75 - 3/Gearbox ==
  Tt : Inport
  Divide : Product  Inputs=*/
  Gear Ratio1 : Constant  Value=gear
  Tt' : Outport
  wires:
  Divide/1 -> Tt'/1
  Tt/1 -> Divide/1
  Gear Ratio1/1 -> Divide/2

== system ieee9bus_wind_farm/GE2.75 - 3/Subsystem ==
  In1 : Inport
  Enable : EnablePort
  Out1 : Outport
  wires:
  In1/1 -> Out1/1

== system ieee9bus_wind_farm/GE2.75 - 3/Subsystem1 ==
  In1 : Inport
  Enable : EnablePort
  Out1 : Outport
  wires:
  In1/1 -> Out1/1

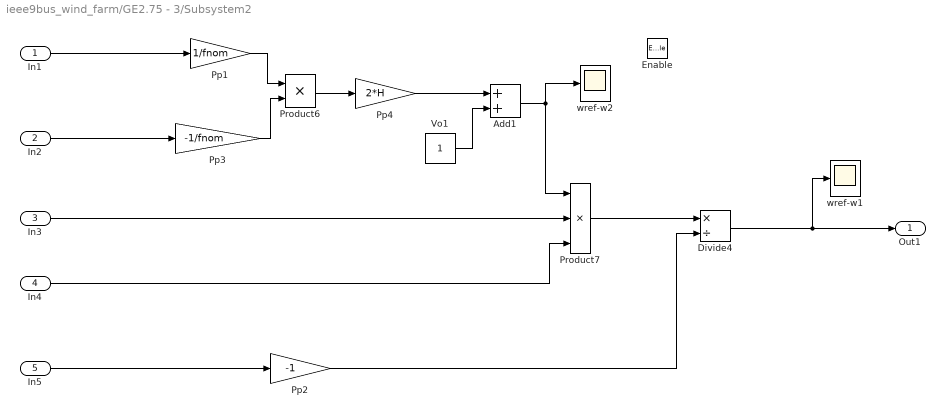
== system ieee9bus_wind_farm/GE2.75 - 3/Subsystem2 ==
  In1 : Inport
  In2 : Inport  Port=2
  In3 : Inport  Port=3
  In4 : Inport  Port=4
  In5 : Inport  Port=5
  Enable : EnablePort
  Add1 : Sum
  Divide4 : Product  Inputs=*/
  Pp1 : Gain  Gain=1/fnom
  Pp2 : Gain  Gain=-1
  Pp3 : Gain  Gain=-1/fnom
  Pp4 : Gain  Gain=2*H
  Product6 : Product
  Product7 : Product  Inputs=3
  Vo1 : Constant
  wref-w1 : Scope
  wref-w2 : Scope
  Out1 : Outport
  wires:
  Pp2/1 -> Divide4/2
  Pp4/1 -> Add1/1
  In1/1 -> Pp1/1
  Divide4/1 -> Out1/1, wref-w1/1
  In4/1 -> Product7/3
  Product7/1 -> Divide4/1
  Product6/1 -> Pp4/1
  Add1/1 -> wref-w2/1, Product7/1
  Vo1/1 -> Add1/2
  Pp1/1 -> Product6/1
  In5/1 -> Pp2/1
  In3/1 -> Product7/2
  In2/1 -> Pp3/1
  Pp3/1 -> Product6/2

== system ieee9bus_wind_farm/GE2.75 - 3/pitch angle controller ==
  wr : Inport
  Constant1 : Constant  Value=1735/1500  SampleTime=Ts
  pitch angle controller : Subsystem
  Beta : Outport
  wires:
  wr/1 -> pitch angle controller/1(wg)
  pitch angle controller/1(pitch) -> Beta/1
  Constant1/1 -> pitch angle controller/2(Ref)

== system ieee9bus_wind_farm/Gen 1/B//2 ==
  R2-1 : powerlib/Elements/Series RLC Branch  LConnTagsString=__new0  RConnTagsString=__new0  BranchType=R  Resistance=10000000000  Inductance=1e-3  SetiL0=off  InitialCurrent=0  Capacitance=1000000*Cbase  Setx0=off  InitialVoltage=0  Measurements=None
  R2-2 : powerlib/Elements/Series RLC Branch  LConnTagsString=__new0  RConnTagsString=__new0  BranchType=R  Resistance=10000000000  Inductance=1e-3  SetiL0=off  InitialCurrent=0  Capacitance=1000000*Cbase  Setx0=off  InitialVoltage=0  Measurements=None
  R2-32 : powerlib/Elements/Series RLC Branch  LConnTagsString=__new0  RConnTagsString=__new0  BranchType=R  Resistance=10000000000  Inductance=1e-3  SetiL0=off  InitialCurrent=0  Capacitance=1000000*Cbase  Setx0=off  InitialVoltage=0  Measurements=None
  Conn1 : PMIOPort  Port=1  Side=Right
  Conn2 : PMIOPort  Port=2  Side=Right
  Conn3 : PMIOPort  Port=3  Side=Right
  connections:
  R2-1/LConn1 -- Conn2/RConn1
  R2-1/RConn1 -- R2-32/RConn1 -- R2-2/RConn1
  R2-32/LConn1 -- Conn1/RConn1
  R2-2/LConn1 -- Conn3/RConn1

== system ieee9bus_wind_farm/Gen 3/B//2 ==
  R2-1 : powerlib/Elements/Series RLC Branch  LConnTagsString=__new0  RConnTagsString=__new0  BranchType=R  Resistance=10000000000  Inductance=1e-3  SetiL0=off  InitialCurrent=0  Capacitance=1000000*Cbase  Setx0=off  InitialVoltage=0  Measurements=None
  R2-2 : powerlib/Elements/Series RLC Branch  LConnTagsString=__new0  RConnTagsString=__new0  BranchType=R  Resistance=10000000000  Inductance=1e-3  SetiL0=off  InitialCurrent=0  Capacitance=1000000*Cbase  Setx0=off  InitialVoltage=0  Measurements=None
  R2-32 : powerlib/Elements/Series RLC Branch  LConnTagsString=__new0  RConnTagsString=__new0  BranchType=R  Resistance=10000000000  Inductance=1e-3  SetiL0=off  InitialCurrent=0  Capacitance=1000000*Cbase  Setx0=off  InitialVoltage=0  Measurements=None
  Conn1 : PMIOPort  Port=1  Side=Right
  Conn2 : PMIOPort  Port=2  Side=Right
  Conn3 : PMIOPort  Port=3  Side=Right
  connections:
  R2-1/LConn1 -- Conn2/RConn1
  R2-1/RConn1 -- R2-32/RConn1 -- R2-2/RConn1
  R2-32/LConn1 -- Conn1/RConn1
  R2-2/LConn1 -- Conn3/RConn1

== system ieee9bus_wind_farm/Gen2/B//2 ==
  R2-1 : powerlib/Elements/Series RLC Branch  LConnTagsString=__new0  RConnTagsString=__new0  BranchType=R  Resistance=10000000000  Inductance=1e-3  SetiL0=off  InitialCurrent=0  Capacitance=1000000*Cbase  Setx0=off  InitialVoltage=0  Measurements=None
  R2-2 : powerlib/Elements/Series RLC Branch  LConnTagsString=__new0  RConnTagsString=__new0  BranchType=R  Resistance=10000000000  Inductance=1e-3  SetiL0=off  InitialCurrent=0  Capacitance=1000000*Cbase  Setx0=off  InitialVoltage=0  Measurements=None
  R2-32 : powerlib/Elements/Series RLC Branch  LConnTagsString=__new0  RConnTagsString=__new0  BranchType=R  Resistance=10000000000  Inductance=1e-3  SetiL0=off  InitialCurrent=0  Capacitance=1000000*Cbase  Setx0=off  InitialVoltage=0  Measurements=None
  Conn1 : PMIOPort  Port=1  Side=Right
  Conn2 : PMIOPort  Port=2  Side=Right
  Conn3 : PMIOPort  Port=3  Side=Right
  connections:
  R2-1/LConn1 -- Conn2/RConn1
  R2-1/RConn1 -- R2-32/RConn1 -- R2-2/RConn1
  R2-32/LConn1 -- Conn1/RConn1
  R2-2/LConn1 -- Conn3/RConn1

== system ieee9bus_wind_farm/Line  5-4/B//1 ==
  Ground : powerlib/Elements/Ground  LConnTagsString=a
  R2-1 : powerlib/Elements/Series RLC Branch  LConnTagsString=__new0  RConnTagsString=__new0  BranchType=C  Resistance=1  Inductance=1e-3  SetiL0=off  InitialCurrent=0  Capacitance=Cbase*0.088  Setx0=off  InitialVoltage=0  Measurements=None
  R2-2 : powerlib/Elements/Series RLC Branch  LConnTagsString=__new0  RConnTagsString=__new0  BranchType=C  Resistance=1  Inductance=1e-3  SetiL0=off  InitialCurrent=0  Capacitance=Cbase*0.088  Setx0=off  InitialVoltage=0  Measurements=None
  R2-3 : powerlib/Elements/Series RLC Branch  LConnTagsString=__new0  RConnTagsString=__new0  BranchType=C  Resistance=1  Inductance=1e-3  SetiL0=off  InitialCurrent=0  Capacitance=Cbase*0.088  Setx0=off  InitialVoltage=0  Measurements=None
  Conn1 : PMIOPort  Port=1  Side=Right
  Conn2 : PMIOPort  Port=2  Side=Right
  Conn3 : PMIOPort  Port=3  Side=Right
  connections:
  R2-2/LConn1 -- Conn1/RConn1
  R2-3/RConn1 -- Ground/LConn1 -- R2-2/RConn1 -- R2-1/RConn1
  R2-3/LConn1 -- Conn3/RConn1
  R2-1/LConn1 -- Conn2/RConn1

== system ieee9bus_wind_farm/Line  5-4/B//2 ==
  Ground : powerlib/Elements/Ground  LConnTagsString=a
  R2-1 : powerlib/Elements/Series RLC Branch  LConnTagsString=__new0  RConnTagsString=__new0  BranchType=C  Resistance=1  Inductance=1e-3  SetiL0=off  InitialCurrent=0  Capacitance=Cbase*0.088  Setx0=off  InitialVoltage=0  Measurements=None
  R2-2 : powerlib/Elements/Series RLC Branch  LConnTagsString=__new0  RConnTagsString=__new0  BranchType=C  Resistance=1  Inductance=1e-3  SetiL0=off  InitialCurrent=0  Capacitance=Cbase*0.088  Setx0=off  InitialVoltage=0  Measurements=None
  R2-3 : powerlib/Elements/Series RLC Branch  LConnTagsString=__new0  RConnTagsString=__new0  BranchType=C  Resistance=1  Inductance=1e-3  SetiL0=off  InitialCurrent=0  Capacitance=Cbase*0.088  Setx0=off  InitialVoltage=0  Measurements=None
  Conn1 : PMIOPort  Port=1  Side=Right
  Conn2 : PMIOPort  Port=2  Side=Right
  Conn3 : PMIOPort  Port=3  Side=Right
  connections:
  R2-1/LConn1 -- Conn2/RConn1
  R2-3/LConn1 -- Conn3/RConn1
  R2-2/RConn1 -- R2-3/RConn1 -- R2-1/RConn1 -- Ground/LConn1
  R2-2/LConn1 -- Conn1/RConn1

== system ieee9bus_wind_farm/Line 6-4/B//1 ==
  Ground : powerlib/Elements/Ground  LConnTagsString=a
  R2-1 : powerlib/Elements/Series RLC Branch  LConnTagsString=__new0  RConnTagsString=__new0  BranchType=C  Resistance=1  Inductance=1e-3  SetiL0=off  InitialCurrent=0  Capacitance=Cbase*0.079  Setx0=off  InitialVoltage=0  Measurements=None
  R2-2 : powerlib/Elements/Series RLC Branch  LConnTagsString=__new0  RConnTagsString=__new0  BranchType=C  Resistance=1  Inductance=1e-3  SetiL0=off  InitialCurrent=0  Capacitance=Cbase*0.079  Setx0=off  InitialVoltage=0  Measurements=None
  R2-3 : powerlib/Elements/Series RLC Branch  LConnTagsString=__new0  RConnTagsString=__new0  BranchType=C  Resistance=1  Inductance=1e-3  SetiL0=off  InitialCurrent=0  Capacitance=Cbase*0.079  Setx0=off  InitialVoltage=0  Measurements=None
  Conn1 : PMIOPort  Port=1  Side=Right
  Conn2 : PMIOPort  Port=2  Side=Right
  Conn3 : PMIOPort  Port=3  Side=Right
  connections:
  R2-1/LConn1 -- Conn2/RConn1
  R2-2/LConn1 -- Conn3/RConn1
  R2-2/RConn1 -- R2-3/RConn1 -- Ground/LConn1 -- R2-1/RConn1
  R2-3/LConn1 -- Conn1/RConn1

== system ieee9bus_wind_farm/Line 6-4/B//2 ==
  Ground : powerlib/Elements/Ground  LConnTagsString=a
  R2-1 : powerlib/Elements/Series RLC Branch  LConnTagsString=__new0  RConnTagsString=__new0  BranchType=C  Resistance=1  Inductance=1e-3  SetiL0=off  InitialCurrent=0  Capacitance=Cbase*0.079  Setx0=off  InitialVoltage=0  Measurements=None
  R2-2 : powerlib/Elements/Series RLC Branch  LConnTagsString=__new0  RConnTagsString=__new0  BranchType=C  Resistance=1  Inductance=1e-3  SetiL0=off  InitialCurrent=0  Capacitance=Cbase*0.079  Setx0=off  InitialVoltage=0  Measurements=None
  R2-3 : powerlib/Elements/Series RLC Branch  LConnTagsString=__new0  RConnTagsString=__new0  BranchType=C  Resistance=1  Inductance=1e-3  SetiL0=off  InitialCurrent=0  Capacitance=Cbase*0.079  Setx0=off  InitialVoltage=0  Measurements=None
  Conn1 : PMIOPort  Port=1  Side=Right
  Conn2 : PMIOPort  Port=2  Side=Right
  Conn3 : PMIOPort  Port=3  Side=Right
  connections:
  R2-3/LConn1 -- Conn1/RConn1
  Ground/LConn1 -- R2-2/RConn1 -- R2-1/RConn1 -- R2-3/RConn1
  R2-2/LConn1 -- Conn3/RConn1
  R2-1/LConn1 -- Conn2/RConn1

== system ieee9bus_wind_farm/Line 7-1/B//1 ==
  Ground : powerlib/Elements/Ground  LConnTagsString=a
  R2-1 : powerlib/Elements/Series RLC Branch  LConnTagsString=__new0  RConnTagsString=__new0  BranchType=C  Resistance=1  Inductance=1e-3  SetiL0=off  InitialCurrent=0  Capacitance=Cbase*0.1045  Setx0=off  InitialVoltage=0  Measurements=None
  R2-2 : powerlib/Elements/Series RLC Branch  LConnTagsString=__new0  RConnTagsString=__new0  BranchType=C  Resistance=1  Inductance=1e-3  SetiL0=off  InitialCurrent=0  Capacitance=Cbase*0.1045  Setx0=off  InitialVoltage=0  Measurements=None
  R2-3 : powerlib/Elements/Series RLC Branch  LConnTagsString=__new0  RConnTagsString=__new0  BranchType=C  Resistance=1  Inductance=1e-3  SetiL0=off  InitialCurrent=0  Capacitance=Cbase*0.1045  Setx0=off  InitialVoltage=0  Measurements=None
  Conn1 : PMIOPort  Port=1  Side=Right
  Conn2 : PMIOPort  Port=2  Side=Right
  Conn3 : PMIOPort  Port=3  Side=Right
  connections:
  R2-1/LConn1 -- Conn2/RConn1
  R2-2/LConn1 -- Conn3/RConn1
  R2-3/RConn1 -- Ground/LConn1 -- R2-2/RConn1 -- R2-1/RConn1
  R2-3/LConn1 -- Conn1/RConn1

== system ieee9bus_wind_farm/Line 7-1/B//2 ==
  Ground : powerlib/Elements/Ground  LConnTagsString=a
  R2-1 : powerlib/Elements/Series RLC Branch  LConnTagsString=__new0  RConnTagsString=__new0  BranchType=C  Resistance=1  Inductance=1e-3  SetiL0=off  InitialCurrent=0  Capacitance=Cbase*0.1045  Setx0=off  InitialVoltage=0  Measurements=None
  R2-2 : powerlib/Elements/Series RLC Branch  LConnTagsString=__new0  RConnTagsString=__new0  BranchType=C  Resistance=1  Inductance=1e-3  SetiL0=off  InitialCurrent=0  Capacitance=Cbase*0.1045  Setx0=off  InitialVoltage=0  Measurements=None
  R2-3 : powerlib/Elements/Series RLC Branch  LConnTagsString=__new0  RConnTagsString=__new0  BranchType=C  Resistance=1  Inductance=1e-3  SetiL0=off  InitialCurrent=0  Capacitance=Cbase*0.1045  Setx0=off  InitialVoltage=0  Measurements=None
  Conn1 : PMIOPort  Port=1  Side=Right
  Conn2 : PMIOPort  Port=2  Side=Right
  Conn3 : PMIOPort  Port=3  Side=Right
  connections:
  R2-3/LConn1 -- Conn1/RConn1
  R2-2/RConn1 -- R2-3/RConn1 -- R2-1/RConn1 -- Ground/LConn1
  R2-2/LConn1 -- Conn3/RConn1
  R2-1/LConn1 -- Conn2/RConn1

== system ieee9bus_wind_farm/Line 7-5/B//1 ==
  Ground : powerlib/Elements/Ground  LConnTagsString=a
  R1 : powerlib/Elements/Series RLC Branch  LConnTagsString=__new0  RConnTagsString=__new0  BranchType=C  Resistance=1  Inductance=1e-3  SetiL0=off  InitialCurrent=0  Capacitance=Cbase*0.153  Setx0=off  InitialVoltage=0  Measurements=None
  R2 : powerlib/Elements/Series RLC Branch  LConnTagsString=__new0  RConnTagsString=__new0  BranchType=C  Resistance=1  Inductance=1e-3  SetiL0=off  InitialCurrent=0  Capacitance=Cbase*0.153  Setx0=off  InitialVoltage=0  Measurements=None
  R3 : powerlib/Elements/Series RLC Branch  LConnTagsString=__new0  RConnTagsString=__new0  BranchType=C  Resistance=1  Inductance=1e-3  SetiL0=off  InitialCurrent=0  Capacitance=Cbase*0.153  Setx0=off  InitialVoltage=0  Measurements=None
  Conn1 : PMIOPort  Port=1  Side=Right
  Conn2 : PMIOPort  Port=2  Side=Right
  Conn3 : PMIOPort  Port=3  Side=Right
  connections:
  R2/LConn1 -- Conn1/RConn1
  Ground/LConn1 -- R2/RConn1 -- R1/RConn1 -- R3/RConn1
  R3/LConn1 -- Conn3/RConn1
  R1/LConn1 -- Conn2/RConn1

== system ieee9bus_wind_farm/Line 7-5/B//2 ==
  Ground : powerlib/Elements/Ground  LConnTagsString=a
  R1 : powerlib/Elements/Series RLC Branch  LConnTagsString=__new0  RConnTagsString=__new0  BranchType=C  Resistance=1  Inductance=1e-3  SetiL0=off  InitialCurrent=0  Capacitance=Cbase*0.153  Setx0=off  InitialVoltage=0  Measurements=None
  R2 : powerlib/Elements/Series RLC Branch  LConnTagsString=__new0  RConnTagsString=__new0  BranchType=C  Resistance=1  Inductance=1e-3  SetiL0=off  InitialCurrent=0  Capacitance=Cbase*0.153  Setx0=off  InitialVoltage=0  Measurements=None
  R3 : powerlib/Elements/Series RLC Branch  LConnTagsString=__new0  RConnTagsString=__new0  BranchType=C  Resistance=1  Inductance=1e-3  SetiL0=off  InitialCurrent=0  Capacitance=Cbase*0.153  Setx0=off  InitialVoltage=0  Measurements=None
  Conn1 : PMIOPort  Port=1  Side=Right
  Conn2 : PMIOPort  Port=2  Side=Right
  Conn3 : PMIOPort  Port=3  Side=Right
  connections:
  R1/LConn1 -- Conn2/RConn1
  R3/LConn1 -- Conn3/RConn1
  R2/RConn1 -- R3/RConn1 -- Ground/LConn1 -- R1/RConn1
  R2/LConn1 -- Conn1/RConn1

== system ieee9bus_wind_farm/Line 7-8/B//1 ==
  Ground : powerlib/Elements/Ground  LConnTagsString=a
  R2-1 : powerlib/Elements/Series RLC Branch  LConnTagsString=__new0  RConnTagsString=__new0  BranchType=C  Resistance=1  Inductance=1e-3  SetiL0=off  InitialCurrent=0  Capacitance=Cbase*0.0745  Setx0=off  InitialVoltage=0  Measurements=None
  R2-2 : powerlib/Elements/Series RLC Branch  LConnTagsString=__new0  RConnTagsString=__new0  BranchType=C  Resistance=1  Inductance=1e-3  SetiL0=off  InitialCurrent=0  Capacitance=Cbase*0.0745  Setx0=off  InitialVoltage=0  Measurements=None
  R2-3 : powerlib/Elements/Series RLC Branch  LConnTagsString=__new0  RConnTagsString=__new0  BranchType=C  Resistance=1  Inductance=1e-3  SetiL0=off  InitialCurrent=0  Capacitance=Cbase*0.0745  Setx0=off  InitialVoltage=0  Measurements=None
  Conn1 : PMIOPort  Port=1  Side=Right
  Conn2 : PMIOPort  Port=2  Side=Right
  Conn3 : PMIOPort  Port=3  Side=Right
  connections:
  R2-3/LConn1 -- Conn1/RConn1
  R2-2/RConn1 -- R2-3/RConn1 -- Ground/LConn1 -- R2-1/RConn1
  R2-2/LConn1 -- Conn3/RConn1
  R2-1/LConn1 -- Conn2/RConn1

== system ieee9bus_wind_farm/Line 7-8/B//2 ==
  Ground : powerlib/Elements/Ground  LConnTagsString=a
  R2-1 : powerlib/Elements/Series RLC Branch  LConnTagsString=__new0  RConnTagsString=__new0  BranchType=C  Resistance=1  Inductance=1e-3  SetiL0=off  InitialCurrent=0  Capacitance=Cbase*0.0745  Setx0=off  InitialVoltage=0  Measurements=None
  R2-2 : powerlib/Elements/Series RLC Branch  LConnTagsString=__new0  RConnTagsString=__new0  BranchType=C  Resistance=1  Inductance=1e-3  SetiL0=off  InitialCurrent=0  Capacitance=Cbase*0.0745  Setx0=off  InitialVoltage=0  Measurements=None
  R2-3 : powerlib/Elements/Series RLC Branch  LConnTagsString=__new0  RConnTagsString=__new0  BranchType=C  Resistance=1  Inductance=1e-3  SetiL0=off  InitialCurrent=0  Capacitance=Cbase*0.0745  Setx0=off  InitialVoltage=0  Measurements=None
  Conn1 : PMIOPort  Port=1  Side=Right
  Conn2 : PMIOPort  Port=2  Side=Right
  Conn3 : PMIOPort  Port=3  Side=Right
  connections:
  R2-1/LConn1 -- Conn2/RConn1
  R2-2/LConn1 -- Conn3/RConn1
  Ground/LConn1 -- R2-2/RConn1 -- R2-1/RConn1 -- R2-3/RConn1
  R2-3/LConn1 -- Conn1/RConn1

== system ieee9bus_wind_farm/Line 9-6/B//1 ==
  Ground : powerlib/Elements/Ground  LConnTagsString=a
  R2-1 : powerlib/Elements/Series RLC Branch  LConnTagsString=__new0  RConnTagsString=__new0  BranchType=C  Resistance=1  Inductance=1e-3  SetiL0=off  InitialCurrent=0  Capacitance=Cbase*0.179  Setx0=off  InitialVoltage=0  Measurements=None
  R2-2 : powerlib/Elements/Series RLC Branch  LConnTagsString=__new0  RConnTagsString=__new0  BranchType=C  Resistance=1  Inductance=1e-3  SetiL0=off  InitialCurrent=0  Capacitance=Cbase*0.179  Setx0=off  InitialVoltage=0  Measurements=None
  R2-3 : powerlib/Elements/Series RLC Branch  LConnTagsString=__new0  RConnTagsString=__new0  BranchType=C  Resistance=1  Inductance=1e-3  SetiL0=off  InitialCurrent=0  Capacitance=Cbase*0.179  Setx0=off  InitialVoltage=0  Measurements=None
  Conn1 : PMIOPort  Port=1  Side=Right
  Conn2 : PMIOPort  Port=2  Side=Right
  Conn3 : PMIOPort  Port=3  Side=Right
  connections:
  R2-1/LConn1 -- Conn2/RConn1
  R2-2/LConn1 -- Conn3/RConn1
  R2-2/RConn1 -- Ground/LConn1 -- R2-3/RConn1 -- R2-1/RConn1
  R2-3/LConn1 -- Conn1/RConn1

== system ieee9bus_wind_farm/Line 9-6/B//2 ==
  Ground : powerlib/Elements/Ground  LConnTagsString=a
  R2-1 : powerlib/Elements/Series RLC Branch  LConnTagsString=__new0  RConnTagsString=__new0  BranchType=C  Resistance=1  Inductance=1e-3  SetiL0=off  InitialCurrent=0  Capacitance=Cbase*0.179  Setx0=off  InitialVoltage=0  Measurements=None
  R2-2 : powerlib/Elements/Series RLC Branch  LConnTagsString=__new0  RConnTagsString=__new0  BranchType=C  Resistance=1  Inductance=1e-3  SetiL0=off  InitialCurrent=0  Capacitance=Cbase*0.179  Setx0=off  InitialVoltage=0  Measurements=None
  R2-3 : powerlib/Elements/Series RLC Branch  LConnTagsString=__new0  RConnTagsString=__new0  BranchType=C  Resistance=1  Inductance=1e-3  SetiL0=off  InitialCurrent=0  Capacitance=Cbase*0.179  Setx0=off  InitialVoltage=0  Measurements=None
  Conn1 : PMIOPort  Port=1  Side=Right
  Conn2 : PMIOPort  Port=2  Side=Right
  Conn3 : PMIOPort  Port=3  Side=Right
  connections:
  R2-3/LConn1 -- Conn1/RConn1
  R2-3/RConn1 -- R2-2/RConn1 -- R2-1/RConn1 -- Ground/LConn1
  R2-2/LConn1 -- Conn3/RConn1
  R2-1/LConn1 -- Conn2/RConn1

== system ieee9bus_wind_farm/GE2.75 - 3/pitch angle controller/pitch angle controller ==
  wg : Inport
  Ref : Inport  Port=2
  "0-pitch_max " : Saturate  UpperLimit=27  LowerLimit=0  SampleTime=Ts
  Discrete PID Controller : simulink/Continuous/PID Controller  Controller=PI  TimeDomain=Discrete-time  SampleTime=Ts  IntegratorMethod=Forward Euler  FilterMethod=Forward Euler  Form=Parallel  UseFilter=on  ControllerParametersSource=internal  P=200  I=25  D=0  N=100  InitialConditionSource=internal  InitialConditionForIntegrator=0  InitialConditionForFilter=0  ExternalReset=none  ZeroCross=off  LimitOutput=on  UpperSaturationLimit=27  LowerSaturationLimit=0  LinearizeAsGain=off  AntiWindupMode=clamping  Kb=1  TrackingMode=off  Kt=1  PParamMin=[]  PParamMax=[]  IParamMin=[]  IParamMax=[]  DParamMin=[]  DParamMax=[]  NParamMin=[]  NParamMax=[]  KbParamMin=[]  KbParamMax=[]  KtParamMin=[]  KtParamMax=[]  POutMin=[]  POutMax=[]  IOutMin=[]  IOutMax=[]  DOutMin=[]  DOutMax=[]  NOutMin=[]  NOutMax=[]  KbOutMin=[]  KbOutMax=[]  KtOutMin=[]  KtOutMax=[]  IntegratorOutMin=[]  IntegratorOutMax=[]  FilterOutMin=[]  FilterOutMax=[]  SumOutMin=[]  SumOutMax=[]  SumI1OutMin=[]  SumI1OutMax=[]  SumI2OutMin=[]  SumI2OutMax=[]  SumI3OutMin=[]  SumI3OutMax=[]  SumDOutMin=[]  SumDOutMax=[]  SaturationOutMin=[]  SaturationOutMax=[]  IntegratorContinuousStateAttributes=''  IntegratorStateMustResolveToSignalObject=off  IntegratorRTWStateStorageClass=Auto  FilterContinuousStateAttributes=''  FilterStateMustResolveToSignalObject=off  FilterRTWStateStorageClass=Auto  DifferentiatorICPrevScaledInput=0  DifferentiatorOutMin=[]  DifferentiatorOutMax=[]
  Rate Limiter : RateLimiter  RisingSlewLimit=10  FallingSlewLimit=-10
  Sum3 : Sum  Inputs=|+-  SampleTime=Ts
  t=Pitch_time_constant1 : powerlib_extras/Discrete  Control Blocks/Discrete 1st-Order Filter  FilterType=Lowpass  Tc=0.02  Ts=Ts  Initialize=on  Vac_Init=[0.8 -25 60]*0  Vdc_Init=0  PlotResponse=off  param1=[1 500 0.1]
  pitch : Outport
  wires:
  Discrete PID Controller/1 -> Rate Limiter/1
  t=Pitch_time_constant1/1 -> pitch/1
  "0-pitch_max "/1 -> t=Pitch_time_constant1/1
  Rate Limiter/1 -> "0-pitch_max "/1
  Ref/1 -> Sum3/2
  wg/1 -> Sum3/1
  Sum3/1 -> Discrete PID Controller/1

== matlab function ieee9bus_wind_farm/GE2.75 - 3/MATLAB Function1 ==
  data: u input; B input; Cp output
function Cp = fcn(u,B)

c1 = 0.5176;
c2 = 116;
c3 = 0.4; 
c4 = 5;
c5 = 21;
c6 = 0.0068;

i =u;

li = 1/((1/(i+0.08*B))-(0.035/(B^3+1)));

Cp = c1*((c2/li-c3*B-c4)*exp(-c5/li))+c6*i;

end
